simulink model "simu_depth"  (R2020b)
settings: Solver=ode1  StartTime=0.0  StopTime=20  FixedStep=1/330*3  RelTol=1e-3
values from neighbouring files (symbols this model uses):
  conIN = [Pixels.signals.values(1,:)'; 1./depo(1)']    [depth_simulations_turtle.m]
settings Model: Creator=Rayane  LastModifiedBy=rayane
settings DebuggingCC: ArithmeticOperatorsInVariantConditions=warning
settings SFSimCC: CustomCodeUndefinedFunction=UseInterfaceOnly

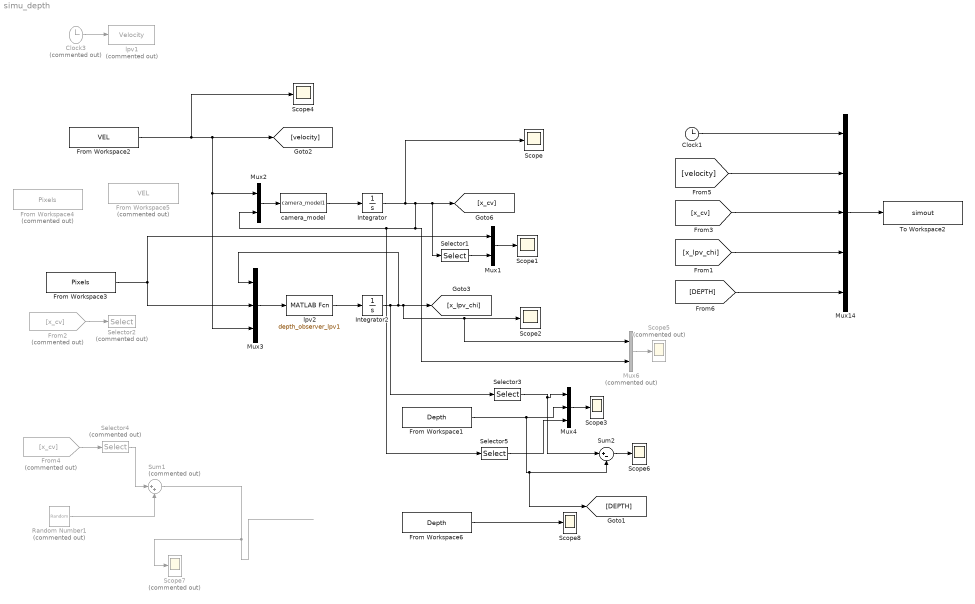
== system simu_depth ==
  Clock1 : Clock
  Clock3 : Clock  Commented=on
  From Workspace1 : FromWorkspace  VariableName=Depth  SampleTime=-1
  From Workspace2 : FromWorkspace  VariableName=VEL  SampleTime=-1
  From Workspace3 : FromWorkspace  VariableName=Pixels  SampleTime=-1
  From Workspace4 : FromWorkspace  Commented=on  VariableName=Pixels  SampleTime=-1
  From Workspace5 : FromWorkspace  Commented=on  VariableName=VEL  SampleTime=-1
  From Workspace6 : FromWorkspace  VariableName=Depth  SampleTime=-1
  From2 : From  Commented=on  GotoTag=x_cv
  From4 : From  Commented=on  GotoTag=x_cv
  Integrator : Integrator  InitialCondition=conIN
  Integrator2 : Integrator  InitialCondition=[0 0 10]
  Mux1 : Mux  Inputs=2
  Mux14 : Mux  Inputs=5
  Mux2 : Mux  Inputs=2
  Mux3 : Mux  Inputs=3
  Mux4 : Mux  Inputs=3
  Mux6 : Mux  Commented=on  Inputs=2
  Random Number1 : RandomNumber  Commented=on  Variance=.01
  Scope{,1..4,6,8} (7 alike) : Scope
  Scope5 : Scope  Commented=on
  Scope7 : Scope  Commented=on
  Selector1 : Selector  InputPortWidth=3  IndexOptions=Index vector (dialog)  Indices=[1,2]  OutputSizes=1
  Selector2 : Selector  Commented=on  InputPortWidth=3  IndexOptions=Index vector (dialog)  Indices=[1 2]  OutputSizes=1
  Selector3 : Selector  InputPortWidth=3  IndexOptions=Index vector (dialog)  Indices=3  OutputSizes=1
  Selector4 : Selector  Commented=on  InputPortWidth=3  IndexOptions=Index vector (dialog)  Indices=[1 2]  OutputSizes=1
  Selector5 : Selector  InputPortWidth=3  IndexOptions=Index vector (dialog)  Indices=3  OutputSizes=1
  Sum1 : Sum  Commented=on  Inputs=|++
  Sum2 : Sum  Inputs=|+-
  To Workspace2 : ToWorkspace  VariableName=simout  SaveFormat=Timeseries  SampleTime=-1
  camera_model : MATLABFcn  MATLABFcn=camera_model1
  lpv1 : MATLABFcn  Commented=on  MATLABFcn=Velocity
  lpv2 : MATLABFcn  MATLABFcn=depth_observer_lpv1
  wires:
  Mux2/1 -> camera_model/1
  camera_model/1 -> Integrator/1
  Mux14/1 -> To Workspace2/1
  Clock1/1 -> Mux14/1
  [velocity] -> Mux14/2
  [x_cv] -> Mux14/3
  Mux3/1 -> lpv2/1
  lpv2/1 -> Integrator2/1
  From Workspace2/1 -> Scope4/1, Mux3/3, Mux2/1, [velocity]
  Integrator2/1 -> Selector3/1, Mux3/1, [x_lpv_chi], Mux6/1, Scope2/1
  Mux6/1 -> Scope5/1
  [x_lpv_chi] -> Mux14/4
  Mux1/1 -> Scope1/1
  Selector1/1 -> Mux1/2
  From Workspace1/1 -> [DEPTH], Sum2/2, Mux4/2
  Mux4/1 -> Scope3/1
  Selector3/1 -> Sum2/1, Mux4/1
  Clock3/1 -> lpv1/1
  Sum1/1 -> Scope7/1
  Random Number1/1 -> Sum1/2
  Selector4/1 -> Sum1/1
  From4/1 -> Selector4/1
  Selector5/1 -> Mux4/3
  Integrator/1 -> Scope/1, Selector1/1, [x_cv], Selector5/1, Mux2/2, Mux6/2
  From2/1 -> Selector2/1
  From Workspace3/1 -> Mux1/1, Mux3/2
  Sum2/1 -> Scope6/1
  [DEPTH] -> Mux14/5
  From Workspace6/1 -> Scope8/1
